simulink model "Planta_completa_controle_velocidade"  (R2023b)
settings: Solver=FixedStepAuto  StartTime=0.0  StopTime=7  FixedStep=T  RelTol=1e-3
model workspace (MAT data in the model file):
  B = 0.0928996133407
  Cmn = 479.991198073
  I = 3000
  Ian = 260.13143483
  J = 0.56
  Kf = 1.91586963478
  La = 0.0014
  N = 3000
  Pele = 104052.573932
  Pmec = 95000
  Ra = 0.08
  T = 0.00175
  Te = 0.0175
  Tm = 6.02801217209
  Vn = 400
  Wn = 197.920296
libraries: simulink x3
settings Model: Creator=USER  LastModifiedBy=USER

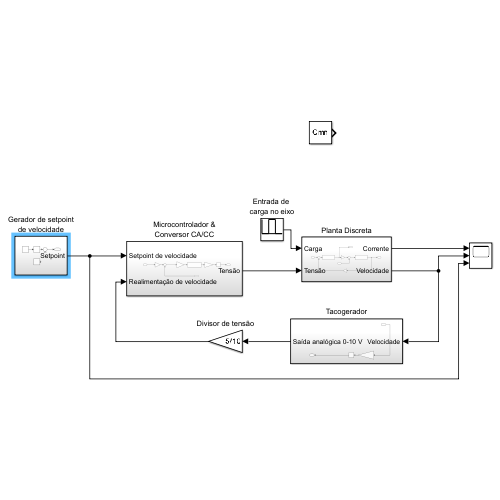
[thumbnail: Simulink's stored preview of the top-level diagram]
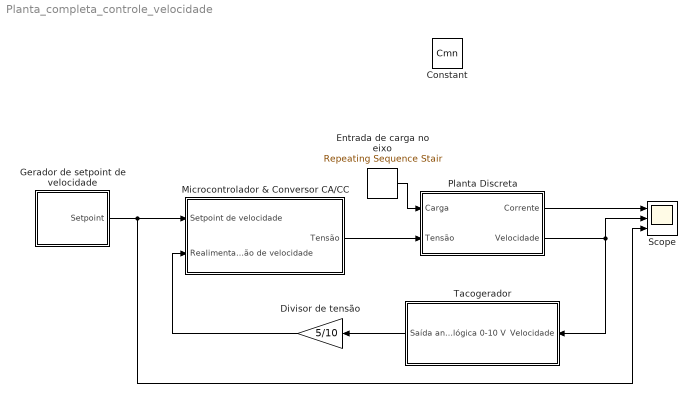
== system Planta_completa_controle_velocidade ==
  Constant : Constant  Value=Cmn
  Divisor de tensão : Gain  Gain=5/10
  Entrada de carga no eixo : simulink/Sources/Repeating Sequence Stair  OutValues=[0, Cmn, 0].'  tsamp=1143 * T  OutMin=[]  OutMax=[]  OutDataTypeStr=double  OutputDataTypeScalingMode=double  OutDataType=fixdt(0,8)  ConRadixGroup=Best Precision: Vector-wise  OutScaling=2^-12
  Gerador de setpoint de velocidade : Subsystem
  Microcontrolador & Conversor CA/CC : Subsystem
  Planta Discreta : Subsystem
  Scope : Scope  NumInputPorts=3
  Tacogerador : Subsystem
  wires:
  Planta Discreta/2(Velocidade) -> Tacogerador/1(Velocidade), Scope/2
  Tacogerador/1(Saída analógica 0-10 V) -> Divisor de tensão/1
  Planta Discreta/1(Corrente) -> Scope/1
  Divisor de tensão/1 -> Microcontrolador & Conversor CA/CC/2(Realimentação de velocidade)
  Microcontrolador & Conversor CA/CC/1(Tensão) -> Planta Discreta/2(Tensão)
  Gerador de setpoint de velocidade/1(Setpoint) -> Scope/3, Microcontrolador & Conversor CA/CC/1(Setpoint de velocidade)
  Entrada de carga no eixo/1 -> Planta Discreta/1(Carga)

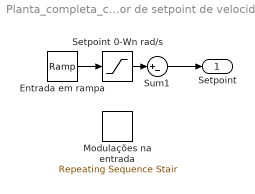
== system Planta_completa_controle_velocidade/Gerador de setpoint de velocidade ==
  Entrada em rampa : simulink/Sources/Ramp  slope=Wn*20  start=0  InitialOutput=0
  Modulações na entrada : simulink/Sources/Repeating Sequence Stair  OutValues=[0 50 -50].'  tsamp=1143 * T  OutMin=[]  OutMax=[]  OutDataTypeStr=double  OutputDataTypeScalingMode=double  OutDataType=fixdt(0,8)  ConRadixGroup=Best Precision: Vector-wise  OutScaling=2^-12
  Setpoint 0-Wn rad/s : Saturate  UpperLimit=Wn
  Sum1 : Sum  Inputs=|+-
  Setpoint : Outport
  wires:
  Setpoint 0-Wn rad/s/1 -> Sum1/1
  Entrada em rampa/1 -> Setpoint 0-Wn rad/s/1
  Sum1/1 -> Setpoint/1

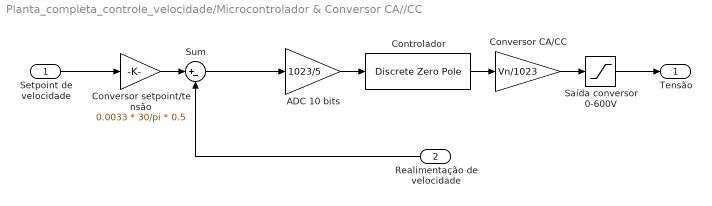
== system Planta_completa_controle_velocidade/Microcontrolador & Conversor CA//CC ==
  Setpoint de velocidade : Inport
  Realimentação de velocidade : Inport  Port=2
  "ADC 10 bits " : Gain  Gain=1023/5
  Controlador : DiscreteZeroPole  Zeros=[0.9]  Poles=[1]  Gain=0.1  SampleTime=-1
  Conversor setpoint/tensão : Gain  Gain=0.0033 * 30/pi * 0.5
  Conversor CA/CC : Gain  Gain=Vn/1023
  Saída conversor 0-600V : Saturate  UpperLimit=600  LowerLimit=0
  Sum : Sum  Inputs=|+-
  Tensão : Outport
  wires:
  Sum/1 -> "ADC 10 bits "/1
  Conversor CA/CC/1 -> Saída conversor 0-600V/1
  Realimentação de velocidade/1 -> Sum/2
  Conversor setpoint/tensão/1 -> Sum/1
  Controlador/1 -> Conversor CA/CC/1
  Setpoint de velocidade/1 -> Conversor setpoint/tensão/1
  "ADC 10 bits "/1 -> Controlador/1
  Saída conversor 0-600V/1 -> Tensão/1

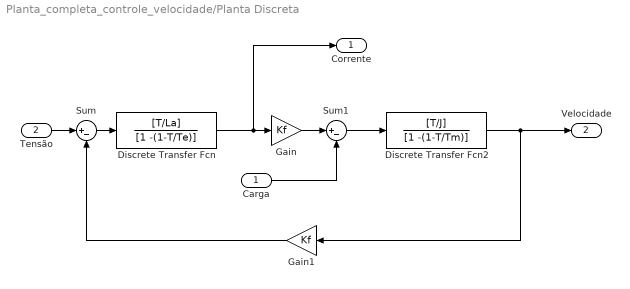
== system Planta_completa_controle_velocidade/Planta Discreta ==
  Carga : Inport
  Tensão : Inport  Port=2
  Discrete Transfer Fcn : DiscreteTransferFcn  Numerator=[T/La]  Denominator=[1 -(1-T/Te)]
  Discrete Transfer Fcn2 : DiscreteTransferFcn  Numerator=[T/J]  Denominator=[1 -(1-T/Tm)]
  Gain : Gain  Gain=Kf
  Gain1 : Gain  Gain=Kf
  Sum : Sum  Inputs=|+-
  Sum1 : Sum  Inputs=|+-
  Corrente : Outport
  Velocidade : Outport  Port=2
  wires:
  Discrete Transfer Fcn/1 -> Gain/1, Corrente/1
  Carga/1 -> Sum1/2
  Tensão/1 -> Sum/1
  Sum1/1 -> Discrete Transfer Fcn2/1
  Gain/1 -> Sum1/1
  Discrete Transfer Fcn2/1 -> Gain1/1, Velocidade/1
  Sum/1 -> Discrete Transfer Fcn/1
  Gain1/1 -> Sum/2

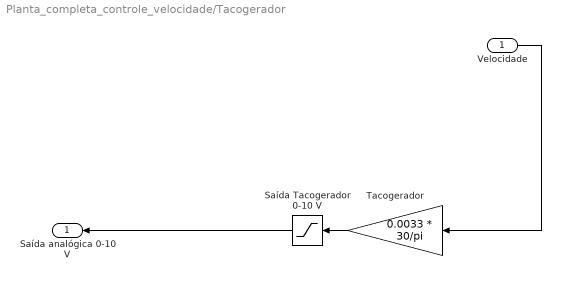
== system Planta_completa_controle_velocidade/Tacogerador ==
  Velocidade : Inport
  Saída Tacogerador 0-10 V : Saturate  UpperLimit=10  LowerLimit=0
  Tacogerador : Gain  Gain=0.0033 * 30/pi
  Saída analógica 0-10 V : Outport
  wires:
  Tacogerador/1 -> Saída Tacogerador 0-10 V/1
  Velocidade/1 -> Tacogerador/1
  Saída Tacogerador 0-10 V/1 -> Saída analógica 0-10 V/1
